simulink model "Zyklus_V3"  (R2020b)
settings: Solver=FixedStepAuto  StartTime=0.0  StopTime=1800  FixedStep=1  RelTol=1e-3
values from neighbouring files (symbols this model uses):
  em =     [ASM_Kennfeld.mat]
  M_achse = [0:5:215]    [Ansteuerung.m]
  n_achse = [0:200:12800]'    [Ansteuerung.m]
  schalt_M = [ schalt_M B]'    [Ansteuerung.m]
  schalt_v = [0:1:140]'    [Ansteuerung.m]
  Wltp_t = [1:1800]'    [Ansteuerung.m]
  Wltp_v = [0;0;0;0;0;0;0;0;0;0;0;0.0555555555555556;0.472222222222222;1.50000000000000;2.75000000000000;3.63888888888889;4.69444444444444;6.02777777777778;7.22222222222222;7.63888888888889;7.80555555555556;7.86111111111111;8;8.08333333333333;8.55555555555556;8.86111111111111;9.47222222222222;10.1666666666667;10.8611111111111;11.4722222222222;11.8055555555556;12.0277777777778;12.1944444444444;12.333333333333 ...(+26189 chars)    [Ansteuerung.m]
settings Model: Creator=Til  LastModifiedBy=kusno

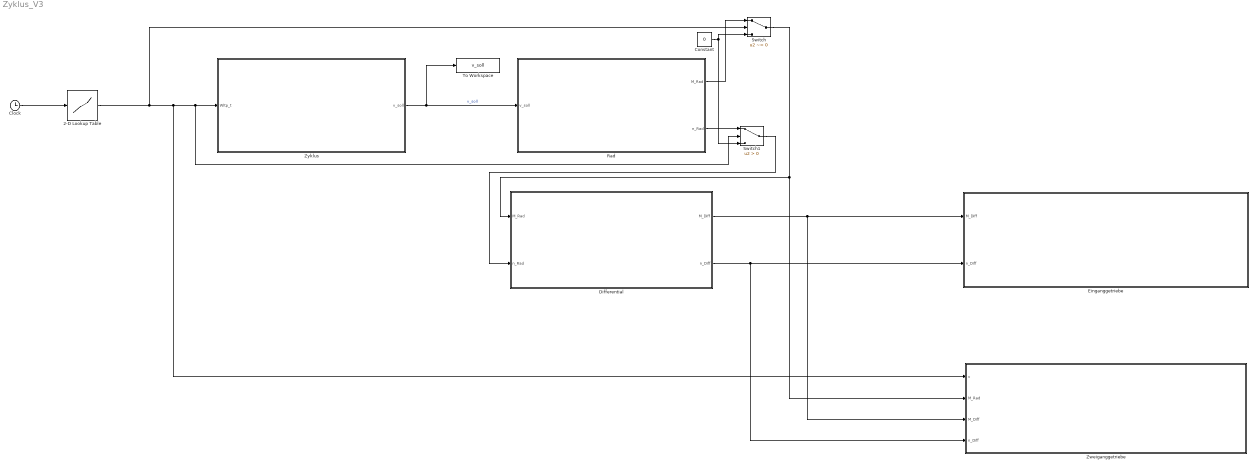
== system Zyklus_V3 ==
  2-D Lookup Table : Lookup_n-D  NumberOfTableDimensions=1  BreakpointsForDimension1=Wltp_t  BreakpointsForDimension2=[1:3]  Table=Wltp_v  InternalRulePriority=Speed  RndMeth=Simplest  InputSameDT=on
  Clock : Clock
  Constant : Constant  Value=0
  Differential : Subsystem
  Einganggetriebe : Subsystem
  Rad : Subsystem
  Switch : Switch  Criteria=u2 ~= 0
  Switch1 : Switch  Criteria=u2 > Threshold
  To Workspace : ToWorkspace  VariableName=v_soll  SaveFormat=Timeseries  SampleTime=-1
  Zweiganggetriebe : Subsystem
  Zyklus : Subsystem
  wires:
  2-D Lookup Table/1 -> Switch/2, Zweiganggetriebe/1(v), Switch1/2, Zyklus/1(Wltp_t)
  Zyklus/1(v_soll) -> To Workspace/1, Rad/1(v_soll)  "v_soll"
  Clock/1 -> 2-D Lookup Table/1
  Differential/1(M_Diff) -> Zweiganggetriebe/3(M_Diff), Einganggetriebe/1(M_Diff)
  Differential/2(n_Diff) -> Zweiganggetriebe/4(n_Diff), Einganggetriebe/2(n_Diff)
  Switch/1 -> Zweiganggetriebe/2(M_Rad), Differential/1(M_Rad)
  Rad/1(M_Rad) -> Switch/1
  Constant/1 -> Switch1/3, Switch/3
  Rad/2(n_Rad) -> Switch1/1
  Switch1/1 -> Differential/2(n_Rad)

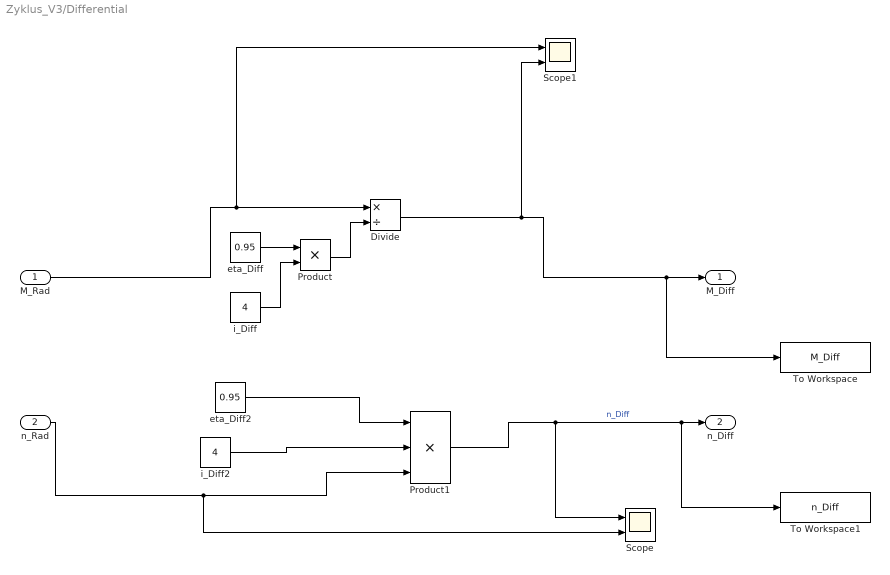
== system Zyklus_V3/Differential ==
  M_Rad : Inport
  n_Rad : Inport  Port=2
  Divide : Product  Inputs=*/
  Product : Product
  Product1 : Product  Inputs=3
  Scope : Scope  NumInputPorts=2
  Scope1 : Scope  NumInputPorts=2
  To Workspace : ToWorkspace  VariableName=M_Diff  SaveFormat=Timeseries  SampleTime=-1
  To Workspace1 : ToWorkspace  VariableName=n_Diff  SaveFormat=Timeseries  SampleTime=-1
  eta_Diff : Constant  Value=0.95
  eta_Diff2 : Constant  Value=0.95
  i_Diff : Constant  Value=4
  i_Diff2 : Constant  Value=4
  M_Diff : Outport
  n_Diff : Outport  Port=2
  wires:
  M_Rad/1 -> Scope1/1, Divide/1
  Divide/1 -> Scope1/2, To Workspace/1, M_Diff/1
  eta_Diff/1 -> Product/1
  i_Diff/1 -> Product/2
  Product/1 -> Divide/2
  eta_Diff2/1 -> Product1/1
  i_Diff2/1 -> Product1/2
  n_Rad/1 -> Scope/2, Product1/3
  Product1/1 -> Scope/1, To Workspace1/1, n_Diff/1  "n_Diff"

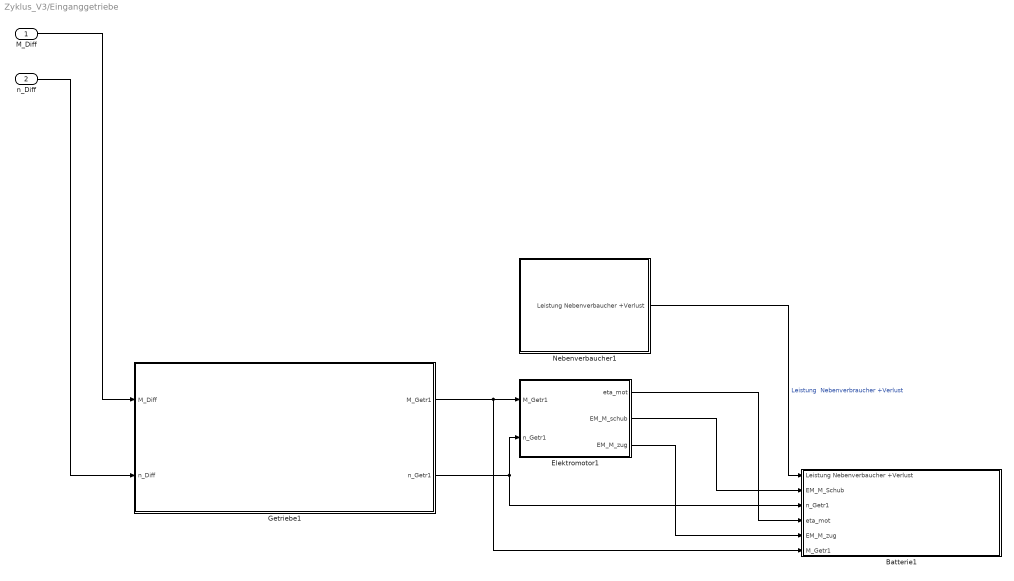
== system Zyklus_V3/Einganggetriebe ==
  M_Diff : Inport
  n_Diff : Inport  Port=2
  Batterie1 : Subsystem
  Elektromotor1 : Subsystem
  Getriebe1 : Subsystem
  Nebenverbaucher1 : Subsystem
  wires:
  Elektromotor1/3(EM_M_zug) -> Batterie1/5(EM_M_zug)
  Elektromotor1/2(EM_M_schub) -> Batterie1/2(EM_M_Schub)
  n_Diff/1 -> Getriebe1/2(n_Diff)
  Nebenverbaucher1/1(Leistung Nebenverbaucher +Verlust) -> Batterie1/1(Leistung Nebenverbaucher +Verlust)  "Leistung  Nebenverbraucher +Verlust"
  Getriebe1/2(n_Getr1) -> Elektromotor1/2(n_Getr1), Batterie1/3(n_Getr1)
  Elektromotor1/1(eta_mot) -> Batterie1/4(eta_mot)
  Getriebe1/1(M_Getr1) -> Batterie1/6(M_Getr1), Elektromotor1/1(M_Getr1)
  M_Diff/1 -> Getriebe1/1(M_Diff)

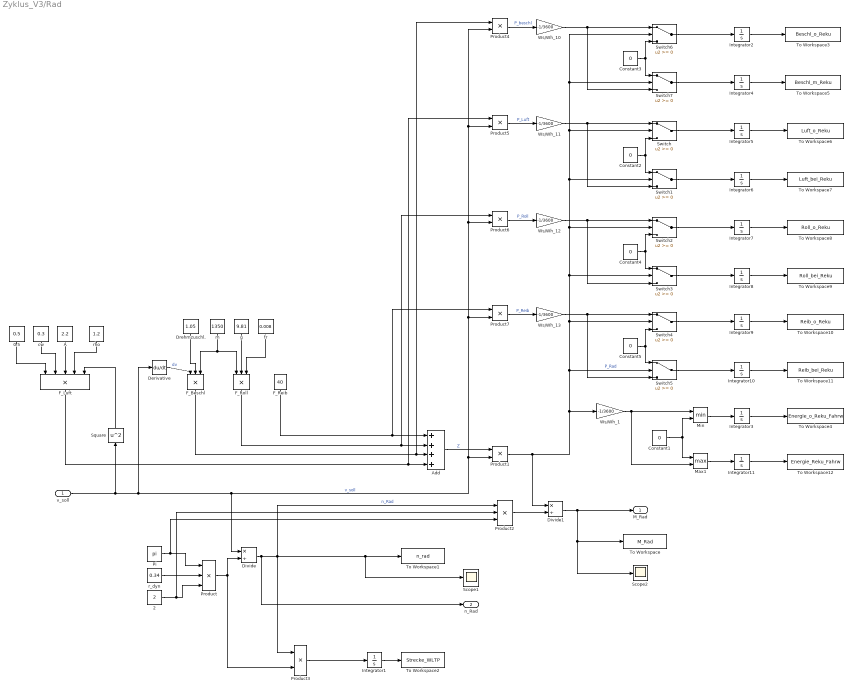
== system Zyklus_V3/Rad ==
  v_soll : Inport
  0.5 : Constant  Value=0.5
  2 : Constant  Value=2
  A : Constant  Value=2.2
  Add : Sum  Inputs=++++
  Constant{1..5} (5 alike) : Constant  Value=0
  Derivative : Derivative
  Divide : Product  Inputs=*/
  Divide1 : Product  Inputs=*/
  Drehmzuschl. : Constant  Value=1.05
  F_Beschl : Product  Inputs=3
  F_Luft : Product  Inputs=5
  F_Reib : Constant  Value=40
  F_Roll : Product  Inputs=3
  Integrator{1..11} (11 alike) : Integrator
  Max1 : MinMax  Function=max  Inputs=2
  Min : MinMax  Inputs=2
  Pi : Constant  Value=pi
  Product : Product  Inputs=3
  Product{1,3..7} (6 alike) : Product
  Product2 : Product  Inputs=3
  Scope1 : Scope
  Scope2 : Scope
  Square : Math  Operator=square  SaturateOnIntegerOverflow=on
  Switch{,1..7} (8 alike) : Switch
  To Workspace : ToWorkspace  VariableName=M_Rad  SaveFormat=Timeseries  SampleTime=-1
  To Workspace1 : ToWorkspace  VariableName=n_rad  SampleTime=-1
      settings: Save2DSignal=2-D array (concatenate along first dimension)
  To Workspace10 : ToWorkspace  VariableName=Reib_o_Reku  SaveFormat=Timeseries  SampleTime=-1
  To Workspace11 : ToWorkspace  VariableName=Reib_bei_Reku  SaveFormat=Timeseries  SampleTime=-1
  To Workspace12 : ToWorkspace  VariableName=Energie_Reku_Fahrw  SaveFormat=Timeseries  SampleTime=-1
  To Workspace2 : ToWorkspace  VariableName=Strecke_WLTP  SampleTime=-1
      settings: Save2DSignal=2-D array (concatenate along first dimension)
  To Workspace3 : ToWorkspace  VariableName=Beschl_o_Reku  SaveFormat=Timeseries  SampleTime=-1
  To Workspace4 : ToWorkspace  VariableName=Energie_o_Reku_Fahrw  SaveFormat=Timeseries  SampleTime=-1
  To Workspace5 : ToWorkspace  VariableName=Beschl_m_Reku  SaveFormat=Timeseries  SampleTime=-1
  To Workspace6 : ToWorkspace  VariableName=Luft_o_Reku  SaveFormat=Timeseries  SampleTime=-1
  To Workspace7 : ToWorkspace  VariableName=Luft_bei_Reku  SaveFormat=Timeseries  SampleTime=-1
  To Workspace8 : ToWorkspace  VariableName=Roll_o_Reku  SaveFormat=Timeseries  SampleTime=-1
  To Workspace9 : ToWorkspace  VariableName=Roll_bei_Reku  SaveFormat=Timeseries  SampleTime=-1
  Ws/Wh_{1,10..13} (5 alike) : Gain  Gain=-1/3600
  cw : Constant  Value=0.3
  fr : Constant  Value=0.008
  g : Constant  Value=9.81
  m : Constant  Value=1350
  r_dyn : Constant  Value=0.34
  rho : Constant  Value=1.2
  M_Rad : Outport
  n_Rad : Outport  Port=2
  wires:
  v_soll/1 -> Product7/2, Product4/2, Product5/2, Product6/2, Product1/2, Divide/1, Derivative/1, Square/1  "v_soll"
  Product/1 -> Product3/2, Divide/2
  Pi/1 -> Product2/3, Product/1
  r_dyn/1 -> Product/2
  2/1 -> Product2/2, Product/3
  Divide/1 -> n_Rad/1, Product3/1, Scope1/1, To Workspace1/1, Product2/1  "n_Rad"
  m/1 -> F_Roll/1, F_Beschl/3
  g/1 -> F_Roll/2
  fr/1 -> F_Roll/3
  Drehmzuschl./1 -> F_Beschl/2
  Derivative/1 -> F_Beschl/1  "dv"
  0.5/1 -> F_Luft/1
  cw/1 -> F_Luft/2
  A/1 -> F_Luft/3
  rho/1 -> F_Luft/4
  F_Reib/1 -> Product7/1, Add/1
  F_Roll/1 -> Product6/1, Add/2
  F_Beschl/1 -> Product4/1, Add/3
  F_Luft/1 -> Product5/1, Add/4
  Add/1 -> Product1/1  "Z"
  Product1/1 -> Switch/2, Switch6/2, Switch7/2, Switch1/2, Switch2/2, Switch3/2, Switch4/2, Switch5/2, Ws/Wh_1/1, Divide1/1  "P_Rad"
  Product2/1 -> Divide1/2
  Divide1/1 -> To Workspace/1, Scope2/1, M_Rad/1
  Square/1 -> F_Luft/5
  Product3/1 -> Integrator1/1
  Integrator1/1 -> To Workspace2/1
  Min/1 -> Integrator3/1
  Constant1/1 -> Max1/1, Min/2
  Integrator3/1 -> To Workspace4/1
  Ws/Wh_1/1 -> Max1/2, Min/1
  Integrator2/1 -> To Workspace3/1
  Integrator4/1 -> To Workspace5/1
  Constant2/1 -> Switch/3, Switch1/1
  Product5/1 -> Ws/Wh_11/1  "P_Luft"
  Constant4/1 -> Switch2/3, Switch3/1
  Product6/1 -> Ws/Wh_12/1  "P_Roll"
  Integrator10/1 -> To Workspace11/1
  Integrator9/1 -> To Workspace10/1
  Constant5/1 -> Switch4/3, Switch5/1
  Product7/1 -> Ws/Wh_13/1  "P_Reib"
  Integrator11/1 -> To Workspace12/1
  Max1/1 -> Integrator11/1
  Switch/1 -> Integrator5/1
  Switch5/1 -> Integrator10/1
  Switch4/1 -> Integrator9/1
  Switch3/1 -> Integrator8/1
  Switch2/1 -> Integrator7/1
  Switch1/1 -> Integrator6/1
  Integrator6/1 -> To Workspace7/1
  Integrator5/1 -> To Workspace6/1
  Integrator7/1 -> To Workspace8/1
  Integrator8/1 -> To Workspace9/1
  Switch7/1 -> Integrator4/1
  Switch6/1 -> Integrator2/1
  Constant3/1 -> Switch6/3, Switch7/1
  Product4/1 -> Ws/Wh_10/1  "P_beschl"
  Ws/Wh_10/1 -> Switch7/3, Switch6/1
  Ws/Wh_11/1 -> Switch1/3, Switch/1
  Ws/Wh_12/1 -> Switch3/3, Switch2/1
  Ws/Wh_13/1 -> Switch5/3, Switch4/1

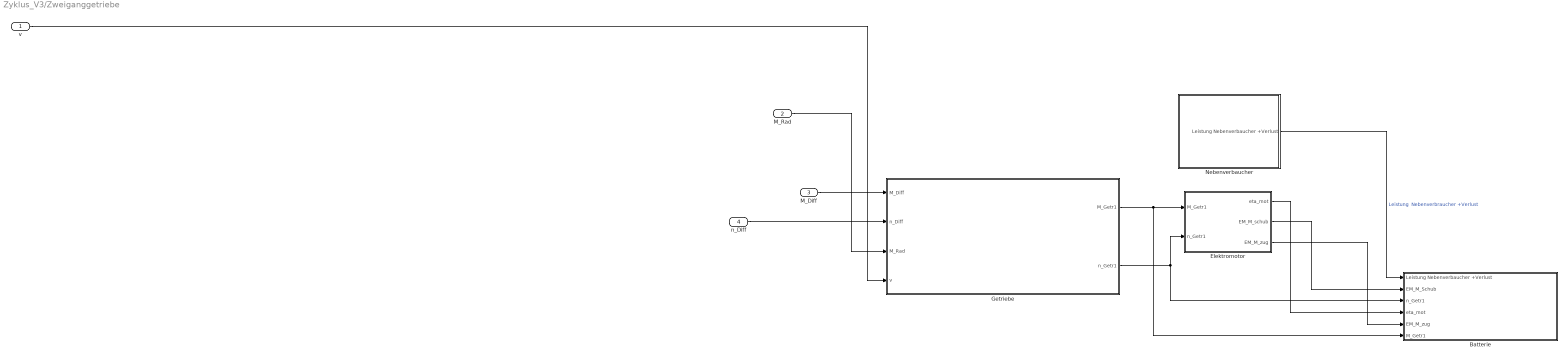
== system Zyklus_V3/Zweiganggetriebe ==
  v : Inport
  M_Rad : Inport  Port=2
  M_Diff : Inport  Port=3
  n_Diff : Inport  Port=4
  Batterie : Subsystem
  Elektromotor : Subsystem
  Getriebe : Subsystem
  Nebenverbaucher : Subsystem
  wires:
  Getriebe/1(M_Getr1) -> Batterie/6(M_Getr1), Elektromotor/1(M_Getr1)
  Nebenverbaucher/1(Leistung Nebenverbaucher +Verlust) -> Batterie/1(Leistung Nebenverbaucher +Verlust)  "Leistung  Nebenverbraucher +Verlust"
  n_Diff/1 -> Getriebe/2(n_Diff)
  M_Rad/1 -> Getriebe/3(M_Rad)
  Elektromotor/1(eta_mot) -> Batterie/4(eta_mot)
  Getriebe/2(n_Getr1) -> Batterie/3(n_Getr1), Elektromotor/2(n_Getr1)
  v/1 -> Getriebe/4(v)
  Elektromotor/2(EM_M_schub) -> Batterie/2(EM_M_Schub)
  Elektromotor/3(EM_M_zug) -> Batterie/5(EM_M_zug)
  M_Diff/1 -> Getriebe/1(M_Diff)

== system Zyklus_V3/Zyklus ==
  Wltp_t : Inport
  v_soll : Outport
  wires:
  Wltp_t/1 -> v_soll/1

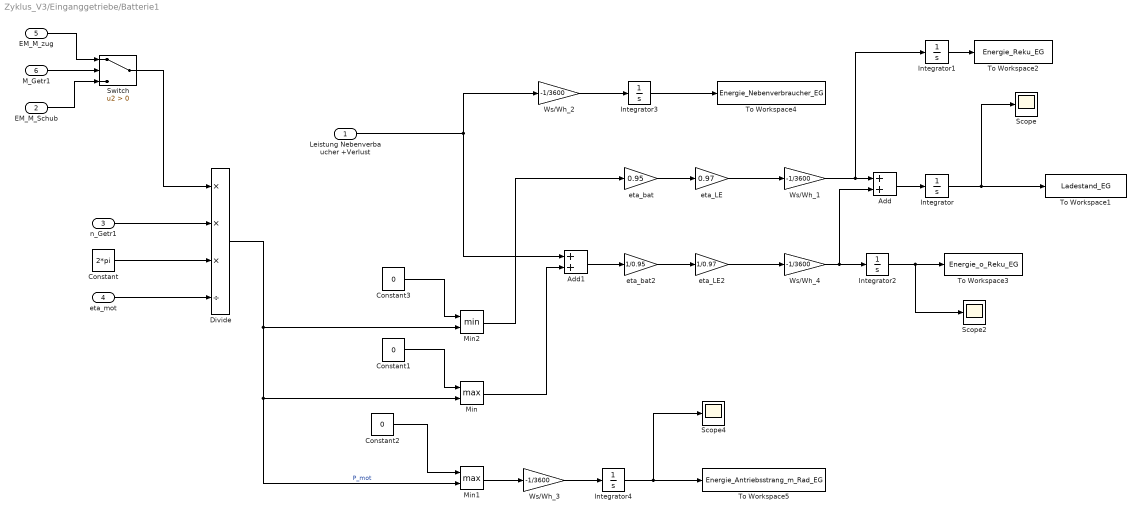
== system Zyklus_V3/Einganggetriebe/Batterie1 ==
  Leistung Nebenverbaucher +Verlust : Inport
  EM_M_Schub : Inport  Port=2
  n_Getr1 : Inport  Port=3
  eta_mot : Inport  Port=4
  EM_M_zug : Inport  Port=5
  M_Getr1 : Inport  Port=6
  Add : Sum
  Add1 : Sum
  Constant : Constant  Value=2*pi
  Constant1 : Constant  Value=0
  Constant2 : Constant  Value=0
  Constant3 : Constant  Value=0
  Divide : Product  Inputs=***/
  Integrator{,1..4} (5 alike) : Integrator
  Min : MinMax  Function=max  Inputs=2
  Min1 : MinMax  Function=max  Inputs=2
  Min2 : MinMax  Inputs=2
  Scope : Scope
  Scope2 : Scope
  Scope4 : Scope
  Switch : Switch  Criteria=u2 > Threshold
  To Workspace1 : ToWorkspace  VariableName=Ladestand_EG  SaveFormat=Timeseries  SampleTime=-1
  To Workspace2 : ToWorkspace  VariableName=Energie_Reku_EG  SaveFormat=Timeseries  SampleTime=-1
  To Workspace3 : ToWorkspace  VariableName=Energie_o_Reku_EG  SaveFormat=Timeseries  SampleTime=-1
  To Workspace4 : ToWorkspace  VariableName=Energie_Nebenverbraucher_EG  SaveFormat=Timeseries  SampleTime=-1
  To Workspace5 : ToWorkspace  VariableName=Energie_Antriebsstrang_m_Rad_EG  SaveFormat=Timeseries  SampleTime=-1
  Ws/Wh_{1..4} (4 alike) : Gain  Gain=-1/3600
  eta_LE : Gain  Gain=0.97
  eta_LE2 : Gain  Gain=1/0.97
  eta_bat : Gain  Gain=0.95
  eta_bat2 : Gain  Gain=1/0.95
  wires:
  n_Getr1/1 -> Divide/2
  eta_mot/1 -> Divide/4
  Constant/1 -> Divide/3
  Divide/1 -> Min2/2, Min1/2, Min/2  "P_mot"
  eta_bat/1 -> eta_LE/1
  Integrator/1 -> Scope/1, To Workspace1/1
  M_Getr1/1 -> Switch/2
  Switch/1 -> Divide/1
  EM_M_zug/1 -> Switch/1
  EM_M_Schub/1 -> Switch/3
  Constant1/1 -> Min/1
  Integrator3/1 -> To Workspace4/1
  Ws/Wh_2/1 -> Integrator3/1
  Constant2/1 -> Min1/1
  Integrator4/1 -> Scope4/1, To Workspace5/1
  Integrator2/1 -> Scope2/1, To Workspace3/1
  Min/1 -> Add1/2
  Leistung Nebenverbaucher +Verlust/1 -> Ws/Wh_2/1, Add1/1
  eta_bat2/1 -> eta_LE2/1
  eta_LE2/1 -> Ws/Wh_4/1
  Ws/Wh_4/1 -> Add/2, Integrator2/1
  Add1/1 -> eta_bat2/1
  Add/1 -> Integrator/1
  eta_LE/1 -> Ws/Wh_1/1
  Ws/Wh_1/1 -> Integrator1/1, Add/1
  Constant3/1 -> Min2/1
  Min2/1 -> eta_bat/1
  Ws/Wh_3/1 -> Integrator4/1
  Min1/1 -> Ws/Wh_3/1
  Integrator1/1 -> To Workspace2/1

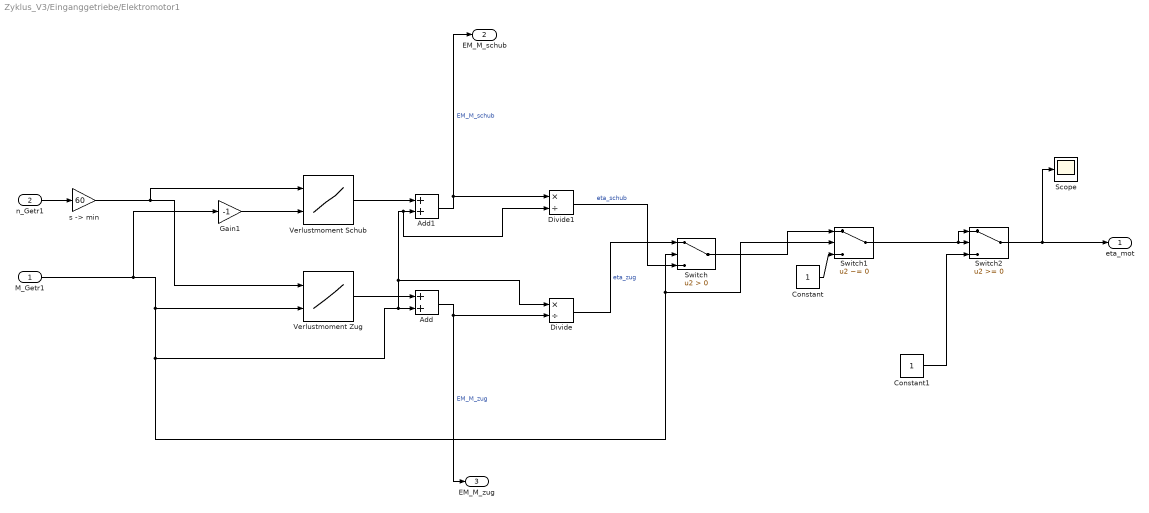
== system Zyklus_V3/Einganggetriebe/Elektromotor1 ==
  M_Getr1 : Inport
  n_Getr1 : Inport  Port=2
  Add : Sum
  Add1 : Sum
  Constant : Constant
  Constant1 : Constant
  Divide : Product  Inputs=*/
  Divide1 : Product  Inputs=*/
  Gain1 : Gain  Gain=-1
  Scope : Scope
  Switch : Switch  Criteria=u2 > Threshold
  Switch1 : Switch  Criteria=u2 ~= 0
  Switch2 : Switch
  Verlustmoment Schub : Lookup_n-D  BreakpointsForDimension1=n_achse  BreakpointsForDimension2=M_achse  Table=em.M_loss_gen_grid  InternalRulePriority=Speed  RndMeth=Simplest  InputSameDT=on
      settings: InputPortMap=u0,u1
  "Verlustmoment Zug " : Lookup_n-D  BreakpointsForDimension1=n_achse  BreakpointsForDimension2=M_achse  Table=em.M_loss_mot_grid  InternalRulePriority=Speed  RndMeth=Simplest  InputSameDT=on
      settings: InputPortMap=u0,u1
  "s -> min" : Gain  Gain=60
  eta_mot : Outport
  EM_M_schub : Outport  Port=2
  EM_M_zug : Outport  Port=3
  wires:
  Verlustmoment Schub/1 -> Add1/1
  M_Getr1/1 -> Gain1/1, "Verlustmoment Zug "/2, Divide1/2, Add1/2, Divide/1, Add/2, Switch/2, Switch1/2
  n_Getr1/1 -> "s -> min"/1
  Divide1/1 -> Switch/3  "eta_schub"
  Add1/1 -> Divide1/1, EM_M_schub/1  "EM_M_schub"
  "Verlustmoment Zug "/1 -> Add/1
  Add/1 -> Divide/2, EM_M_zug/1  "EM_M_zug"
  Divide/1 -> Switch/1  "eta_zug"
  "s -> min"/1 -> Verlustmoment Schub/1, "Verlustmoment Zug "/1
  Gain1/1 -> Verlustmoment Schub/2
  Switch/1 -> Switch1/1
  Constant/1 -> Switch1/3
  Constant1/1 -> Switch2/3
  Switch1/1 -> Switch2/1, Switch2/2
  Switch2/1 -> Scope/1, eta_mot/1

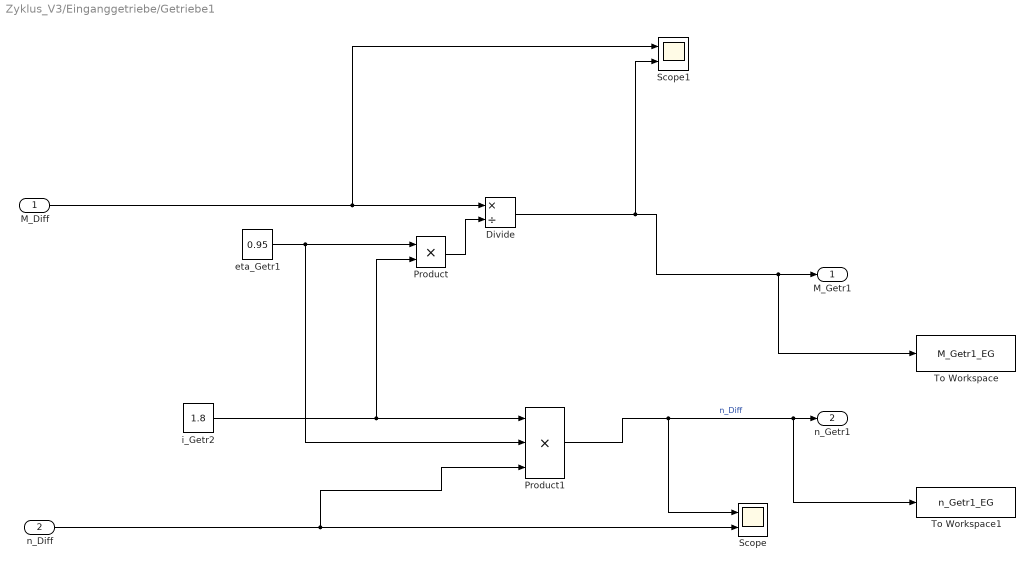
== system Zyklus_V3/Einganggetriebe/Getriebe1 ==
  M_Diff : Inport
  n_Diff : Inport  Port=2
  Divide : Product  Inputs=*/
  Product : Product
  Product1 : Product  Inputs=3
  Scope : Scope  NumInputPorts=2
  Scope1 : Scope  NumInputPorts=2
  To Workspace : ToWorkspace  VariableName=M_Getr1_EG  SaveFormat=Timeseries  SampleTime=-1
  To Workspace1 : ToWorkspace  VariableName=n_Getr1_EG  SaveFormat=Timeseries  SampleTime=-1
  eta_Getr1 : Constant  Value=0.95
  i_Getr2 : Constant  Value=1.8
  M_Getr1 : Outport
  n_Getr1 : Outport  Port=2
  wires:
  Product1/1 -> Scope/1, n_Getr1/1, To Workspace1/1  "n_Diff"
  M_Diff/1 -> Scope1/1, Divide/1
  n_Diff/1 -> Product1/3, Scope/2
  eta_Getr1/1 -> Product1/2, Product/1
  Divide/1 -> Scope1/2, M_Getr1/1, To Workspace/1
  Product/1 -> Divide/2
  i_Getr2/1 -> Product/2, Product1/1

== system Zyklus_V3/Einganggetriebe/Nebenverbaucher1 ==
  Gain : Gain  Gain=1/0.95
  Leistung Nebenverbraucher : Constant  Value=200
  Leistung Nebenverbaucher +Verlust : Outport
  wires:
  Gain/1 -> Leistung Nebenverbaucher +Verlust/1
  Leistung Nebenverbraucher/1 -> Gain/1

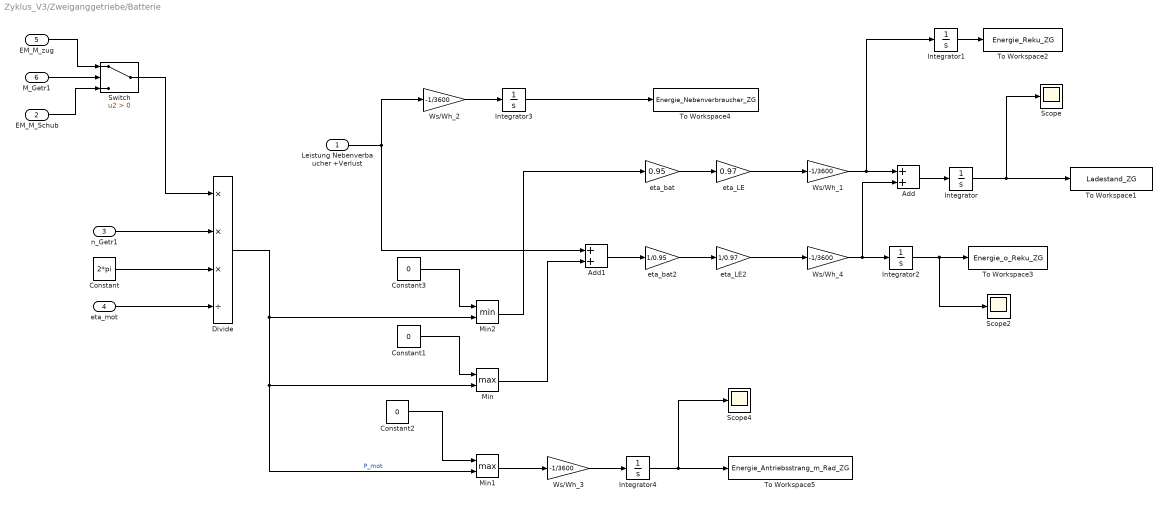
== system Zyklus_V3/Zweiganggetriebe/Batterie ==
  Leistung Nebenverbaucher +Verlust : Inport
  EM_M_Schub : Inport  Port=2
  n_Getr1 : Inport  Port=3
  eta_mot : Inport  Port=4
  EM_M_zug : Inport  Port=5
  M_Getr1 : Inport  Port=6
  Add : Sum
  Add1 : Sum
  Constant : Constant  Value=2*pi
  Constant1 : Constant  Value=0
  Constant2 : Constant  Value=0
  Constant3 : Constant  Value=0
  Divide : Product  Inputs=***/
  Integrator{,1..4} (5 alike) : Integrator
  Min : MinMax  Function=max  Inputs=2
  Min1 : MinMax  Function=max  Inputs=2
  Min2 : MinMax  Inputs=2
  Scope : Scope
  Scope2 : Scope
  Scope4 : Scope
  Switch : Switch  Criteria=u2 > Threshold
  To Workspace1 : ToWorkspace  VariableName=Ladestand_ZG  SaveFormat=Timeseries  SampleTime=-1
  To Workspace2 : ToWorkspace  VariableName=Energie_Reku_ZG  SaveFormat=Timeseries  SampleTime=-1
  To Workspace3 : ToWorkspace  VariableName=Energie_o_Reku_ZG  SaveFormat=Timeseries  SampleTime=-1
  To Workspace4 : ToWorkspace  VariableName=Energie_Nebenverbraucher_ZG  SaveFormat=Timeseries  SampleTime=-1
  To Workspace5 : ToWorkspace  VariableName=Energie_Antriebsstrang_m_Rad_ZG  SaveFormat=Timeseries  SampleTime=-1
  Ws/Wh_{1..4} (4 alike) : Gain  Gain=-1/3600
  eta_LE : Gain  Gain=0.97
  eta_LE2 : Gain  Gain=1/0.97
  eta_bat : Gain  Gain=0.95
  eta_bat2 : Gain  Gain=1/0.95
  wires:
  n_Getr1/1 -> Divide/2
  eta_mot/1 -> Divide/4
  Constant/1 -> Divide/3
  M_Getr1/1 -> Switch/2
  Switch/1 -> Divide/1
  EM_M_zug/1 -> Switch/1
  EM_M_Schub/1 -> Switch/3
  Integrator3/1 -> To Workspace4/1
  Ws/Wh_2/1 -> Integrator3/1
  eta_bat2/1 -> eta_LE2/1
  eta_LE2/1 -> Ws/Wh_4/1
  Add/1 -> Integrator/1
  Add1/1 -> eta_bat2/1
  Constant3/1 -> Min2/1
  Ws/Wh_3/1 -> Integrator4/1
  Integrator/1 -> Scope/1, To Workspace1/1
  Min2/1 -> eta_bat/1
  Constant2/1 -> Min1/1
  Integrator2/1 -> Scope2/1, To Workspace3/1
  eta_LE/1 -> Ws/Wh_1/1
  Min/1 -> Add1/2
  Integrator4/1 -> Scope4/1, To Workspace5/1
  eta_bat/1 -> eta_LE/1
  Constant1/1 -> Min/1
  Leistung Nebenverbaucher +Verlust/1 -> Ws/Wh_2/1, Add1/1
  Divide/1 -> Min1/2, Min/2, Min2/2  "P_mot"
  Ws/Wh_4/1 -> Add/2, Integrator2/1
  Min1/1 -> Ws/Wh_3/1
  Integrator1/1 -> To Workspace2/1
  Ws/Wh_1/1 -> Integrator1/1, Add/1

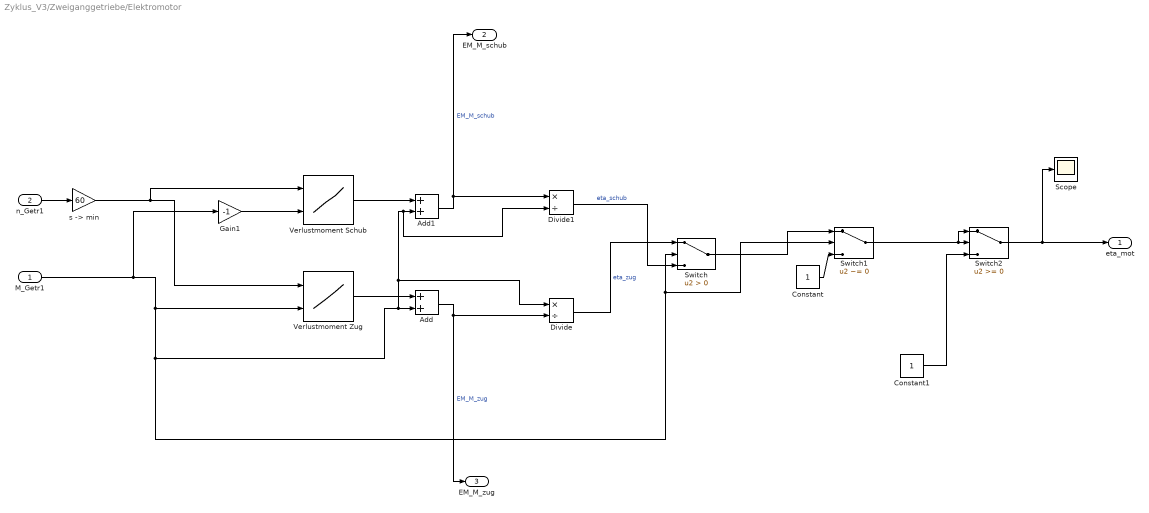
== system Zyklus_V3/Zweiganggetriebe/Elektromotor ==
  M_Getr1 : Inport
  n_Getr1 : Inport  Port=2
  Add : Sum
  Add1 : Sum
  Constant : Constant
  Constant1 : Constant
  Divide : Product  Inputs=*/
  Divide1 : Product  Inputs=*/
  Gain1 : Gain  Gain=-1
  Scope : Scope
  Switch : Switch  Criteria=u2 > Threshold
  Switch1 : Switch  Criteria=u2 ~= 0
  Switch2 : Switch
  Verlustmoment Schub : Lookup_n-D  BreakpointsForDimension1=n_achse  BreakpointsForDimension2=M_achse  Table=em.M_loss_gen_grid  InternalRulePriority=Speed  RndMeth=Simplest  InputSameDT=on
      settings: InputPortMap=u0,u1
  "Verlustmoment Zug " : Lookup_n-D  BreakpointsForDimension1=n_achse  BreakpointsForDimension2=M_achse  Table=em.M_loss_mot_grid  InternalRulePriority=Speed  RndMeth=Simplest  InputSameDT=on
      settings: InputPortMap=u0,u1
  "s -> min" : Gain  Gain=60
  eta_mot : Outport
  EM_M_schub : Outport  Port=2
  EM_M_zug : Outport  Port=3
  wires:
  Verlustmoment Schub/1 -> Add1/1
  M_Getr1/1 -> Gain1/1, "Verlustmoment Zug "/2, Divide1/2, Add1/2, Divide/1, Add/2, Switch/2, Switch1/2
  n_Getr1/1 -> "s -> min"/1
  Divide1/1 -> Switch/3  "eta_schub"
  Add1/1 -> Divide1/1, EM_M_schub/1  "EM_M_schub"
  "Verlustmoment Zug "/1 -> Add/1
  Add/1 -> Divide/2, EM_M_zug/1  "EM_M_zug"
  Divide/1 -> Switch/1  "eta_zug"
  "s -> min"/1 -> Verlustmoment Schub/1, "Verlustmoment Zug "/1
  Gain1/1 -> Verlustmoment Schub/2
  Switch/1 -> Switch1/1
  Constant/1 -> Switch1/3
  Constant1/1 -> Switch2/3
  Switch1/1 -> Switch2/1, Switch2/2
  Switch2/1 -> Scope/1, eta_mot/1

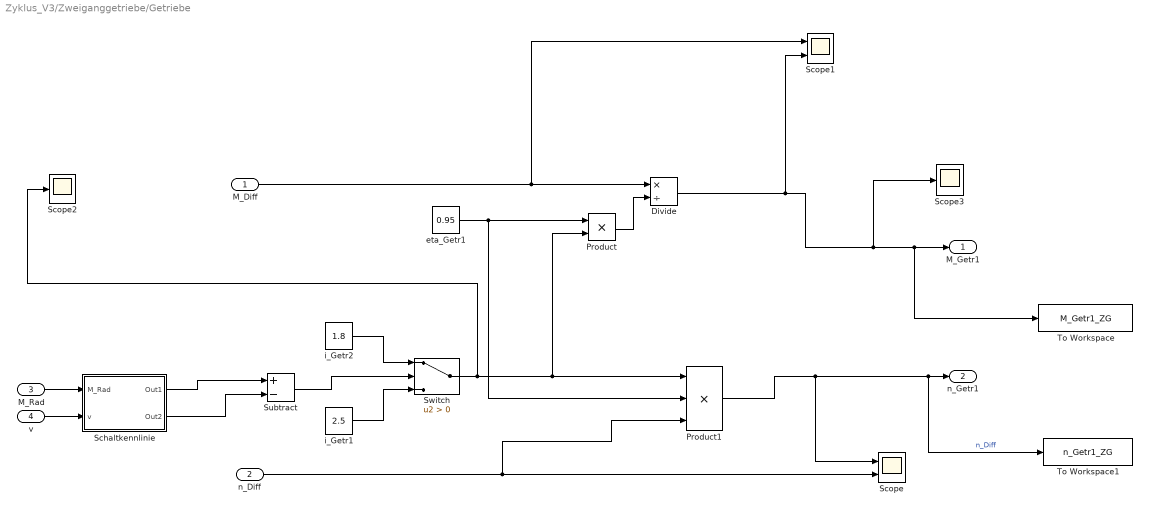
== system Zyklus_V3/Zweiganggetriebe/Getriebe ==
  M_Diff : Inport
  n_Diff : Inport  Port=2
  M_Rad : Inport  Port=3
  v : Inport  Port=4
  Divide : Product  Inputs=*/
  Product : Product
  Product1 : Product  Inputs=3
  Schaltkennlinie : Subsystem
  Scope : Scope  NumInputPorts=2
  Scope1 : Scope  NumInputPorts=2
  Scope2 : Scope
  Scope3 : Scope
  Subtract : Sum  Inputs=+-
  Switch : Switch  Criteria=u2 > Threshold
  To Workspace : ToWorkspace  VariableName=M_Getr1_ZG  SaveFormat=Timeseries  SampleTime=-1
  To Workspace1 : ToWorkspace  VariableName=n_Getr1_ZG  SaveFormat=Timeseries  SampleTime=-1
  eta_Getr1 : Constant  Value=0.95
  i_Getr1 : Constant  Value=2.5
  i_Getr2 : Constant  Value=1.8
  M_Getr1 : Outport
  n_Getr1 : Outport  Port=2
  wires:
  Product1/1 -> Scope/1, n_Getr1/1, To Workspace1/1  "n_Diff"
  M_Diff/1 -> Scope1/1, Divide/1
  n_Diff/1 -> Product1/3, Scope/2
  eta_Getr1/1 -> Product1/2, Product/1
  Divide/1 -> Scope1/2, Scope3/1, M_Getr1/1, To Workspace/1
  Product/1 -> Divide/2
  Switch/1 -> Scope2/1, Product/2, Product1/1
  Subtract/1 -> Switch/2
  i_Getr1/1 -> Switch/3
  i_Getr2/1 -> Switch/1
  M_Rad/1 -> Schaltkennlinie/1(M_Rad)
  v/1 -> Schaltkennlinie/2(v)
  Schaltkennlinie/1(Out1) -> Subtract/1
  Schaltkennlinie/2(Out2) -> Subtract/2

== system Zyklus_V3/Zweiganggetriebe/Nebenverbaucher ==
  Gain : Gain  Gain=1/0.95
  Leistung Nebenverbraucher : Constant  Value=200
  Leistung Nebenverbaucher +Verlust : Outport
  wires:
  Gain/1 -> Leistung Nebenverbaucher +Verlust/1
  Leistung Nebenverbraucher/1 -> Gain/1

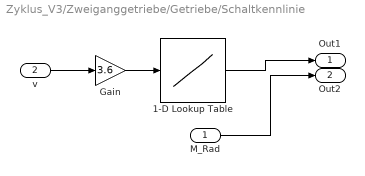
== system Zyklus_V3/Zweiganggetriebe/Getriebe/Schaltkennlinie ==
  M_Rad : Inport
  v : Inport  Port=2
  1-D Lookup Table : Lookup_n-D  NumberOfTableDimensions=1  BreakpointsForDimension1=schalt_v  Table=schalt_M  InternalRulePriority=Speed  RndMeth=Simplest  InputSameDT=on
  Gain : Gain  Gain=3.6
  Out1 : Outport
  Out2 : Outport  Port=2
  wires:
  1-D Lookup Table/1 -> Out1/1
  v/1 -> Gain/1
  Gain/1 -> 1-D Lookup Table/1
  M_Rad/1 -> Out2/1
